simulink model "P5"  (R2020b)
settings: Solver=VariableStepAuto  StartTime=0.0  StopTime=10.0  RelTol=1e-3
settings Model: Creator=ASUS  LastModifiedBy=ASUS

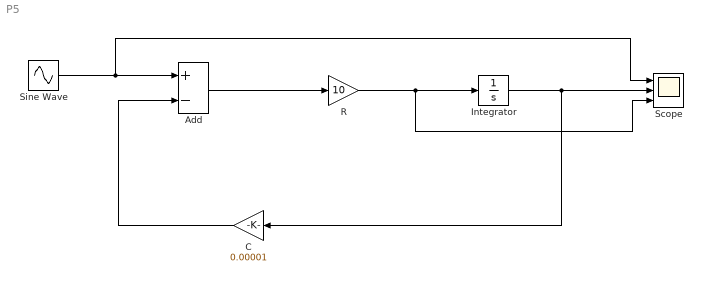
== system P5 ==
  Add : Sum  Inputs=+-
  C : Gain  Gain=0.00001
  Integrator : Integrator
  R : Gain  Gain=10
  Scope : Scope  NumInputPorts=3
  Sine Wave : Sin  Frequency=5  SampleTime=0
  wires:
  Sine Wave/1 -> Scope/1, Add/1
  Add/1 -> R/1
  C/1 -> Add/2
  Integrator/1 -> C/1, Scope/2
  R/1 -> Integrator/1, Scope/3
